simulink model "GA_Sin_NoLin_2"  (R2017a)
settings: Solver=FixedStepAuto  StartTime=0.0  StopTime=4*pi  MaxStep=1e-4  RelTol=1e-6
libraries: powerlib x6, powerlib_meascontrol x3
settings Model: Creator=pagilm  LastModifiedBy=pagilm

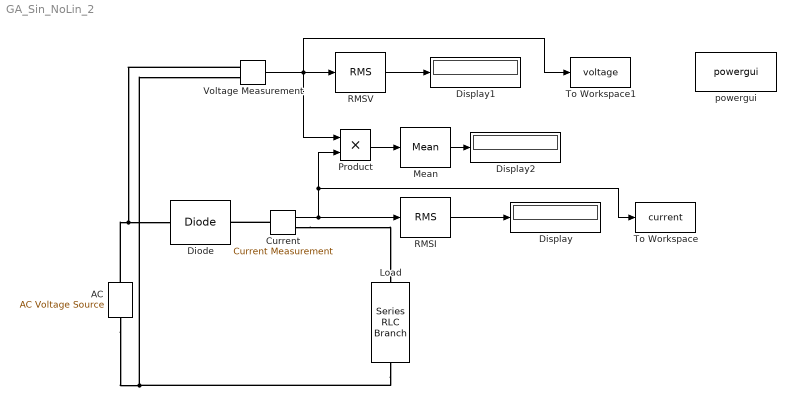
== system GA_Sin_NoLin_2 ==
  AC : powerlib/Electrical Sources/AC Voltage Source  Amplitude=230*sqrt(2)  Phase=0  Frequency=50  SampleTime=0  Measurements=None  BusType=swing  Pref=10e3  Qref=0  Qmin=-inf  Qmax=+inf
  "Current " : powerlib/Measurements/Current Measurement  PhasorSimulation=off  OutputType=Complex  PSBequivalent=0
  Diode : powerlib/Power Electronics/Diode  Ron=0.001  Lon=0  Vf=0.1  IC=0  UseSnubber=0  Rs=500  Cs=250e-9  Measurements=off
  Display : Display
  Display1 : Display
  Display2 : Display
  Load : powerlib/Elements/Series RLC Branch  LConnTagsString=__new0  RConnTagsString=__new0  BranchType=RL  Resistance=1  Inductance=2e-3  SetiL0=off  InitialCurrent=0  Capacitance=1e-6  Setx0=off  InitialVoltage=0  Measurements=None
  Mean : powerlib_meascontrol/Measurements/Mean  Freq=1/2/pi  Vinit=0  Ts=0
  Product : Product
  RMSI : powerlib_meascontrol/Measurements/RMS  TrueRMS=on  Freq=1/2/pi  RMSInit=0  Ts=0
  RMSV : powerlib_meascontrol/Measurements/RMS  TrueRMS=on  Freq=1/2/pi  RMSInit=0  Ts=0
  To Workspace : ToWorkspace  VariableName=current  SaveFormat=Structure With Time  SampleTime=-1
  To Workspace1 : ToWorkspace  VariableName=voltage  SaveFormat=Structure With Time  SampleTime=-1
  Voltage Measurement : powerlib/Measurements/Voltage Measurement  PhasorSimulation=off  OutputType=Complex  PSBequivalent=0
  powergui : powerlib/powergui  Priority=1  SimulationMode=Discrete  SampleTime=50e-6  frequency=60  Iterations=50  frequencyindice=50  Pbase=100e6  ErrMax=1e-4  UnitsV=kV  UnitsW=MW  buscounter=0  FunctionMessages=off  echomessages=off  EnableUseOfTLC=off  CurrentSourceSwitches=off  DisableSnubberDevices=off  DisableRonSwitches=off  DisableVfSwitches=off  DisplayEquations=off  SolverType=Tustin/Backward Euler (TBE)  Interpol=off  ExternalGateDelay=off  methode=off  Ts=100  x0status=blocks  SPID=off  SwTol=0  HookPort=off  RestoreLinks=warning  ResistiveCurrentMeasurement=off  Frange=[0:2:500]  Ylog=off  Xlog=on  ShowGrid=off  save=off  variable=ZData  structure=0  ZoomFFT=off  StartTime=0.0  cycles=1  DisplayStyle=1  fundamental=60  FreqAxis=off  MaxFrequency=1000  frequencyindicesteady=1  RmsSteady=1  display=off
  wires:
  RMSV/1 -> Display1/1
  Product/1 -> Mean/1
  Mean/1 -> Display2/1
  Voltage Measurement/1 -> To Workspace1/1, RMSV/1, Product/1
  "Current "/1 -> To Workspace/1, Product/2, RMSI/1
  RMSI/1 -> Display/1
  connections:
  AC/RConn1 -- Voltage Measurement/LConn1 -- Diode/LConn1
  Load/RConn1 -- AC/LConn1 -- Voltage Measurement/LConn2
  "Current "/LConn1 -- Diode/RConn1
  "Current "/RConn1 -- Load/LConn1
